simulink model "DCservo"  (R2022a)
settings: Solver=FixedStepAuto  StartTime=0.0  StopTime=test_duration  FixedStep=0.002  RelTol=1e-3
InitFcn:
  | model_parameters
values from neighbouring files (symbols this model uses):
  A = [0 0; 1 0]    [model_parameters.m]    (also in model_parameters.mat = [0  0; 1  0])
  afDen = conv(fo,fo)    [model_parameters.m]    (also in model_parameters.mat = [5.10204081633e-05 0.0142857142857 1])
  B = [5*2.25; 0]*max_int10/10    [model_parameters.m]    (also in model_parameters.mat = [576 0])
  C = eye(2)    [model_parameters.m]    (also in model_parameters.mat = [1  0; 0  1])
  coulomb_linear = 0.5    [model_parameters.m]    (also in model_parameters.mat)
  D = [0;0]    [model_parameters.m]    (also in model_parameters.mat = [0 0])
  dead_zone_half_width = 0.3    [model_parameters.m]    (also in model_parameters.mat)
  int_to_volt = volts/max_int10    (= 0.01953125)    [model_parameters.m]    (also in model_parameters.mat)
  linear_friction = 0.12    [model_parameters.m]    (also in model_parameters.mat)
  max_int10 = 2^(n_bits-1)    (= 512)    [model_parameters.m]    (also in model_parameters.mat)
  quad_friction = 0.03    [model_parameters.m]    (also in model_parameters.mat)
  volt_to_int = max_int10/volts    (= 51.2)    [model_parameters.m]    (also in model_parameters.mat)
  volts = 10    [model_parameters.m]    (also in model_parameters.mat)
undefined symbols (not defined in the file or in its folder): sut_nl
libraries: simulink x4, simulink_extras x1
settings Model: Creator=claudio  LastModifiedBy=claudio
settings SolverCC: AlgebraicLoopSolver=TrustRegion
settings DebuggingCC: UnconnectedInputMsg=warning  UnconnectedOutputMsg=warning  UnconnectedLineMsg=warning  SFMachineParentedDataDiag=warning
settings SFSimCC: SimCustomHeaderCode="#include \"controllers.h\""  SimUserIncludeDirs=include
settings SFSimCC: SimUserSources=|
  | src/pos_float.c
  | src/pos_fixed.c

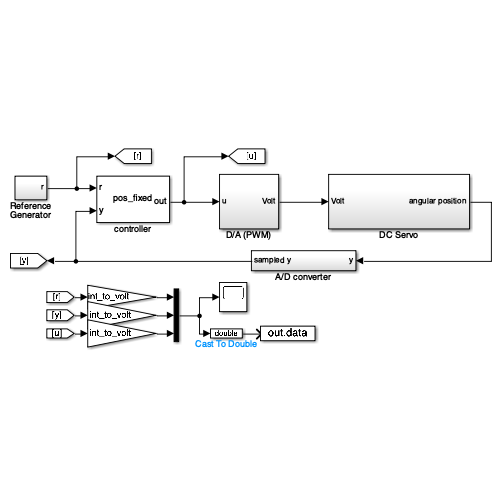
[thumbnail: Simulink's stored preview of the top-level diagram]
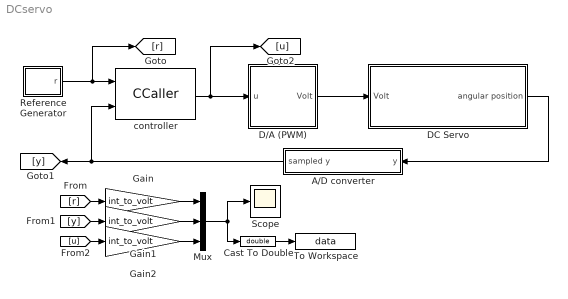
== system DCservo ==
  A/D converter : Subsystem
  Cast To Double : DataTypeConversion  OutDataTypeStr=double  SaturateOnIntegerOverflow=off  RndMeth=Floor
  D/A (PWM) : Subsystem
  "DC Servo " : Subsystem
  Gain : Gain  Gain=int_to_volt
  Gain1 : Gain  Gain=int_to_volt
  Gain2 : Gain  Gain=int_to_volt
  Mux : Mux  Inputs=3
  Reference Generator : Subsystem
  Scope : Scope
  To Workspace : ToWorkspace  VariableName=data  SaveFormat=Timeseries  SampleTime=-1
  controller : CCaller  FunctionName=pos_fixed  PortSpecificationStruct="%)30     .    6 4   8    (     @         %    \"     ,    !     0         %  0 \"0    $    _    07)G3F%M90  4&]R=$YA;64 4V-O<&4     26YD97@     5'EP90      4VEZ90      27-';&]B86P   X    P    !@    @    $          4    (     0    ,    !         !   P!O=70 #@   #     &    \"     0         !0    @    !     P    $         $  # &]U=  .    .     8    (    !          %    \"     $    &     0         0    !@   $]U='!U=   #@   #@    &    \"     8         !0    @    !     0    $         \"0    @               X    X    !@    @    $          4    (     0    4    !         !     %    :6YT,38    .    ,     8    (    !          %    \"     $    !     0         0  $ ,0    X    P    !@    @    ) @        4    (     0    $    !          (  0      #@   #     &    \"     0         !0    @    !     0    $         $  ! '(    .    ,     8    (    !          %    \"     $    !     0         0  $ <@    X    X    !@    @    $          4    (     0    4    !         !     %    26YP=70    .    .     8    (    !@         %    \"     $    !     0         )    \"               #@   #@    &    \"     0         !0    @    !    !0    $         $     4   !I;G0Q-@    X    P    !@    @    $          4    (     0    $    !         !   0 Q    #@   #     &    \"     D\"        !0    @    !     0    $          @ !       .    ,     8    (    !          %    \"     $    !     0         0  $ >0    X    P    !@    @    $          4    (     0    $    !         !   0!Y    #@   #@    &    \"     0         !0    @    !    !0    $         $     4   !);G!U=     X    X    !@    @    &          4    (     0    $    !          D    (            \\#\\.    .     8    (    !          %    \"     $    %     0         0    !0   &EN=#$V    #@   #     &    \"     0         !0    @    !     0    $         $  ! #$    .    ,     8    (    \"0(        %    \"     $    !     0         \"  $"
  wires:
  Gain/1 -> Mux/1
  Gain1/1 -> Mux/2
  Gain2/1 -> Mux/3
  Reference Generator/1(r) -> [r], controller/1
  [r] -> Gain/1
  [y] -> Gain1/1
  [u] -> Gain2/1
  controller/1 -> [u], D/A (PWM)/1(u)
  D/A (PWM)/1(Volt) -> "DC Servo "/1(Volt)
  A/D converter/1(sampled y) -> controller/2, [y]
  "DC Servo "/1(angular position) -> A/D converter/1(y)
  Mux/1 -> Cast To Double/1, Scope/1
  Cast To Double/1 -> To Workspace/1

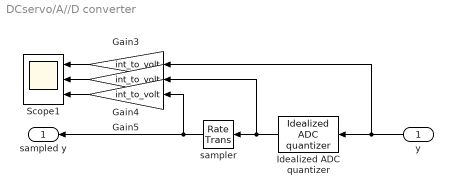
== system DCservo/A//D converter ==
  y : Inport
  Gain3 : Gain  Gain=int_to_volt
  Gain4 : Gain  Gain=int_to_volt
  Gain5 : Gain  Gain=int_to_volt
  Idealized ADC quantizer : simulink_extras/Additional Discrete/Idealized ADC quantizer  NumberOfConverterBits=n_bits  Vmin=-512  Vmax=511  OutputDataType=int16  OutputNegativeValues=on
  Scope1 : Scope  NumInputPorts=3
  sampler : RateTransition  OutPortSampleTime=ctrl_loop_sampling_time
  sampled y : Outport
  wires:
  Gain4/1 -> Scope1/2
  Gain3/1 -> Scope1/1
  sampler/1 -> sampled y/1, Gain5/1
  Idealized ADC quantizer/1 -> Gain4/1, sampler/1
  Gain5/1 -> Scope1/3
  y/1 -> Gain3/1, Idealized ADC quantizer/1

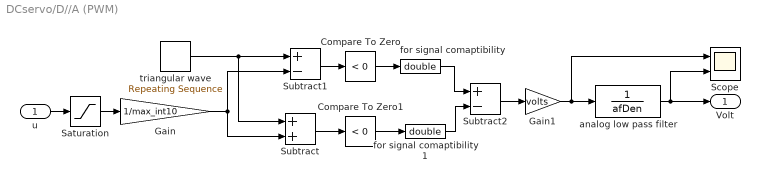
== system DCservo/D//A (PWM) ==
  u : Inport
  Compare To Zero : simulink/Logic and Bit Operations/Compare To Zero  relop=<  OutDataTypeStr=boolean
  Compare To Zero1 : simulink/Logic and Bit Operations/Compare To Zero  relop=<  OutDataTypeStr=boolean
  Gain : Gain  Gain=1/max_int10
  Gain1 : Gain  Gain=volts
  Saturation : Saturate  UpperLimit=511  LowerLimit=-512
  Scope : Scope  NumInputPorts=2
  Subtract : Sum
  Subtract1 : Sum  Inputs=+-
  Subtract2 : Sum  Inputs=+-
  analog low pass filter : TransferFcn  Numerator=1  Denominator=afDen
  for signal comaptibility : DataTypeConversion  OutMin=[-512]  OutMax=[511]  OutDataTypeStr=double  SaturateOnIntegerOverflow=off  RndMeth=Floor
  for signal comaptibility1 : DataTypeConversion  OutMin=[-512]  OutMax=[511]  OutDataTypeStr=double  SaturateOnIntegerOverflow=off  RndMeth=Floor
  triangular wave : simulink/Sources/Repeating Sequence  rep_seq_t=[0 0.01]  rep_seq_y=[0 1]
  Volt : Outport
  wires:
  u/1 -> Saturation/1
  Saturation/1 -> Gain/1
  Subtract1/1 -> Compare To Zero/1
  Subtract2/1 -> Gain1/1
  Compare To Zero1/1 -> for signal comaptibility1/1
  Compare To Zero/1 -> for signal comaptibility/1
  for signal comaptibility/1 -> Subtract2/1
  analog low pass filter/1 -> Volt/1, Scope/2
  Subtract/1 -> Compare To Zero1/1
  for signal comaptibility1/1 -> Subtract2/2
  triangular wave/1 -> Subtract/1, Subtract1/1
  Gain/1 -> Subtract1/2, Subtract/2
  Gain1/1 -> analog low pass filter/1, Scope/1

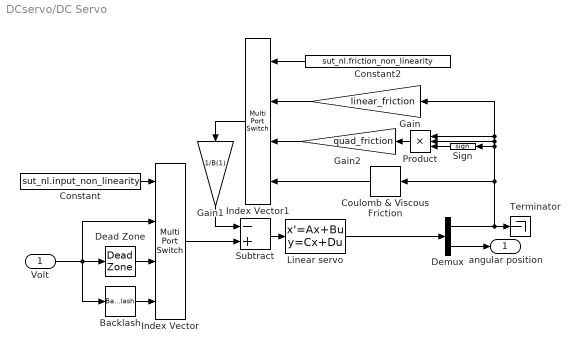
== system DCservo/DC Servo  ==
  Volt : Inport
  Backlash : Backlash  BacklashWidth=deadband_width
  Constant : Constant  Value=sut_nl.input_non_linearity
  Constant2 : Constant  Value=sut_nl.friction_non_linearity
  Coulomb & Viscous Friction : simulink/Discontinuities/Coulomb & Viscous Friction  offset=coulomb_static  gain=coulomb_linear
  Dead Zone : DeadZone  LowerValue=-dead_zone_half_width  UpperValue=dead_zone_half_width
  Demux : Demux  Outputs=2
  Gain : Gain  Gain=linear_friction
  Gain1 : Gain  Gain=1/B(1)
  Gain2 : Gain  Gain=quad_friction
  Index Vector : MultiPortSwitch  DataPortOrder=Zero-based contiguous  zeroidx=on  SaturateOnIntegerOverflow=off  InputSameDT=off
  Index Vector1 : MultiPortSwitch  DataPortOrder=Zero-based contiguous  zeroidx=on  SaturateOnIntegerOverflow=off  InputSameDT=off
  Linear servo : StateSpace  A=A  B=B  C=C  D=D  InitialCondition=[0,0]
  Product : Product  Inputs=3
  Sign : Signum
  Subtract : Sum  Inputs=-+
  Terminator : Terminator
  angular position : Outport
  wires:
  Demux/1 -> Coulomb & Viscous Friction/1, Product/2, Product/1, Gain/1, Sign/1, Terminator/1
  Demux/2 -> angular position/1
  Linear servo/1 -> Demux/1
  Index Vector/1 -> Subtract/2
  Constant/1 -> Index Vector/1
  Volt/1 -> Backlash/1, Index Vector/2, Dead Zone/1
  Dead Zone/1 -> Index Vector/3
  Backlash/1 -> Index Vector/4
  Subtract/1 -> Linear servo/1
  Gain/1 -> Index Vector1/2
  Constant2/1 -> Index Vector1/1
  Index Vector1/1 -> Gain1/1
  Gain1/1 -> Subtract/1
  Gain2/1 -> Index Vector1/3
  Product/1 -> Gain2/1
  Coulomb & Viscous Friction/1 -> Index Vector1/4
  Sign/1 -> Product/3

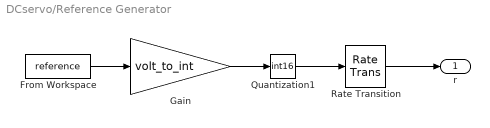
== system DCservo/Reference Generator ==
  From Workspace : FromWorkspace  VariableName=reference  OutDataTypeStr=double  Interpolate=off  OutputAfterFinalValue=Holding final value
  Gain : Gain  Gain=volt_to_int
  Quantization1 : DataTypeConversion  OutMin=[-512]  OutMax=[511]  OutDataTypeStr=int16  SaturateOnIntegerOverflow=off  RndMeth=Floor
  Rate Transition : RateTransition  OutPortSampleTime=ctrl_loop_sampling_time
  r : Outport
  wires:
  Rate Transition/1 -> r/1
  Quantization1/1 -> Rate Transition/1
  From Workspace/1 -> Gain/1
  Gain/1 -> Quantization1/1
